simulink model "fbl_4wd_model_debug"  (R2020b)
settings: Solver=VariableStepAuto  StartTime=0.0  StopTime=1  RelTol=1e-6
values from neighbouring files (symbols this model uses):
  a = 0.37    [main.m]
  b = 0.55    [main.m]
  d0 = 0.18    [main.m]
  fr_act = 0.12    [main.m]
  g = 9.81    [main.m]
  I = 20    [main.m]
  M = [m 0 0; 0 m 0; 0 0 I]    [main.m]
  m = 116    [main.m]
  mu_act = 0.88    [main.m]
  q0 = [0;0;deg2rad(10)]    [main.m]
  q0_dot = [[cos(q0(3)) -sin(q0(3));sin(q0(3)) cos(q0(3))]*[0.5;0.5];-2.2]    [main.m]
  r = 0.2    [main.m]
libraries: simulink x2
settings Model: Creator=sumit  LastModifiedBy=sumit

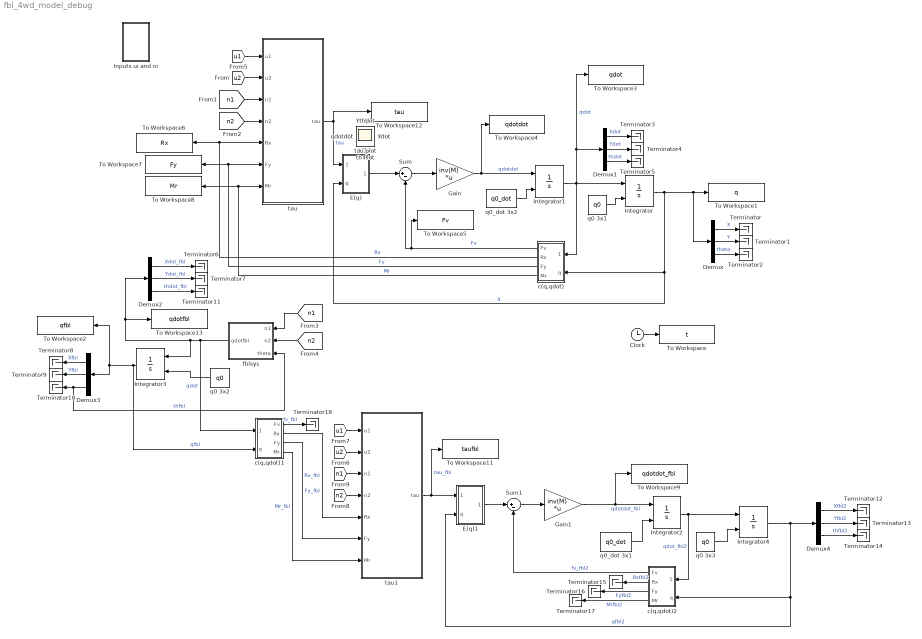
== system fbl_4wd_model_debug ==
  Clock : Clock
  Demux{,1..4} (5 alike) : Demux  Outputs=3
  E(q) : Subsystem
  E(q)1 : Subsystem
  Gain : Gain  Gain=inv(M)  Multiplication=Matrix(K*u) (u vector)
  Gain1 : Gain  Gain=inv(M)  Multiplication=Matrix(K*u) (u vector)
  Inputs ui and ni : Subsystem
  Integrator{,1..4} (5 alike) : Integrator  InitialConditionSource=external
  Sum : Sum  Inputs=|+-
  Sum1 : Sum  Inputs=|+-
  Terminator{,1..18} (19 alike) : Terminator
  To Workspace : ToWorkspace  VariableName=t  SampleTime=-1
  To Workspace1 : ToWorkspace  VariableName=q  SampleTime=-1
  To Workspace11 : ToWorkspace  VariableName=taufbl  SampleTime=-1
  To Workspace12 : ToWorkspace  VariableName=tau  SampleTime=-1
  To Workspace13 : ToWorkspace  VariableName=qdotfbl  SampleTime=-1
  To Workspace2 : ToWorkspace  VariableName=qfbl  SampleTime=-1
  To Workspace3 : ToWorkspace  VariableName=qdot  SampleTime=-1
  To Workspace4 : ToWorkspace  VariableName=qdotdot  SampleTime=-1
  To Workspace5 : ToWorkspace  VariableName=Fv  SampleTime=-1
  To Workspace6 : ToWorkspace  VariableName=Rx  SampleTime=-1
  To Workspace7 : ToWorkspace  VariableName=Fy  SampleTime=-1
  To Workspace8 : ToWorkspace  VariableName=Mr  SampleTime=-1
  To Workspace9 : ToWorkspace  VariableName=qdotdot_fbl  SampleTime=-1
  c(q,qdot) : Subsystem
  c(q,qdot)1 : Subsystem
  c(q,qdot)2 : Subsystem
  fblsys : MATLAB Function  TreatAsAtomicUnit=on
  q0 3x1 : Constant  Value=q0
  q0 3x2 : Constant  Value=q0
  q0 3x3 : Constant  Value=q0
  q0_dot 3x1 : Constant  Value=q0_dot
  q0_dot 3x2 : Constant  Value=q0_dot
  tau : MATLAB Function  TreatAsAtomicUnit=on
  tau1 : MATLAB Function  TreatAsAtomicUnit=on
  Fv : Scope
  Fy : Scope
  Mr : Scope
  Rx : Scope
  X Plot : Scope
  Xdot : Scope
  Y Plot : Scope
  Ydot : Scope
  qdotdot : Scope
  tau plot : Scope
  th Plot : Scope
  thdot : Scope
  wires:
  q0 3x1/1 -> Integrator/2
  q0_dot 3x2/1 -> Integrator1/2
  Gain/1 -> To Workspace4/1, Integrator1/1  "qdotdot"
  Clock/1 -> To Workspace/1
  Integrator/1 -> c(q,qdot)/2(q), E(q)/2(q), Demux/1, To Workspace1/1  "q"
  Sum/1 -> Gain/1
  c(q,qdot)/1(Fv) -> To Workspace5/1, Sum/2  "Fv"
  E(q)/1(Ftau) -> Sum/1
  Demux/1 -> Terminator/1  "X"
  Demux/2 -> Terminator1/1  "Y"
  Demux/3 -> Terminator2/1  "theta"
  Demux1/2 -> Terminator4/1  "Ydot"
  Integrator1/1 -> Integrator/1, c(q,qdot)/1(qdot), To Workspace3/1, Demux1/1  "qdot"
  Demux1/3 -> Terminator5/1  "thdot"
  Demux1/1 -> Terminator3/1  "Xdot"
  tau/1(tau) -> E(q)/1(tau), To Workspace12/1  "tau"
  c(q,qdot)/4(Mr) -> To Workspace8/1, tau/7(Mr)  "Mr"
  c(q,qdot)/3(Fy) -> To Workspace7/1, tau/6(Fy)  "Fy"
  c(q,qdot)/2(Rx) -> To Workspace6/1, tau/5(Rx)  "Rx"
  [n1] -> tau/3(n1)
  [n2] -> tau/4(n2)
  [n1] -> fblsys/1(n1)
  [n2] -> fblsys/2(n2)
  q0 3x2/1 -> Integrator3/2
  Demux3/1 -> Terminator8/1  "Xfbl"
  Integrator3/1 -> c(q,qdot)1/2(q), Demux3/1, To Workspace2/1  "qfbl"
  Demux3/2 -> Terminator9/1  "Yfbl"
  Demux3/3 -> fblsys/3(theta), Terminator10/1  "thfbl"
  Demux2/1 -> Terminator6/1  "Xdot_fbl"
  Demux2/2 -> Terminator7/1  "Ydot_fbl"
  Demux2/3 -> Terminator11/1  "thdot_fbl"
  fblsys/1(qdotfbl) -> Integrator3/1, To Workspace13/1, Demux2/1, c(q,qdot)1/1(qdot)  "qdot"
  c(q,qdot)1/1(Fv) -> Terminator18/1  "fv_fbl"
  c(q,qdot)1/2(Rx) -> tau1/5(Rx)  "Rx_fbl"
  c(q,qdot)1/3(Fy) -> tau1/6(Fy)  "Fy_fbl"
  c(q,qdot)1/4(Mr) -> tau1/7(Mr)  "Mr_fbl"
  [u2] -> tau/2(u2)
  [u1] -> tau/1(u1)
  [u1] -> tau1/1(u1)
  [u2] -> tau1/2(u2)
  [n1] -> tau1/3(n1)
  [n2] -> tau1/4(n2)
  tau1/1(tau) -> To Workspace11/1, E(q)1/1(tau)  "tau_fbl"
  E(q)1/1(Ftau) -> Sum1/1
  Sum1/1 -> Gain1/1
  Gain1/1 -> Integrator2/1, To Workspace9/1  "qdotdot_fbl"
  q0_dot 3x1/1 -> Integrator2/2
  q0 3x3/1 -> Integrator4/2
  Integrator2/1 -> Integrator4/1, c(q,qdot)2/1(qdot)  "qdot_fbl2"
  Integrator4/1 -> E(q)1/2(q), c(q,qdot)2/2(q), Demux4/1  "qfbl2"
  Demux4/1 -> Terminator12/1  "Xfbl2"
  Demux4/2 -> Terminator13/1  "Yfbl2"
  Demux4/3 -> Terminator14/1  "thfbl2"
  c(q,qdot)2/2(Rx) -> Terminator15/1  "Rxfbl2"
  c(q,qdot)2/3(Fy) -> Terminator16/1  "Fyfbl2"
  c(q,qdot)2/4(Mr) -> Terminator17/1  "Mrfbl2"
  c(q,qdot)2/1(Fv) -> Sum1/2  "fv_fbl2"

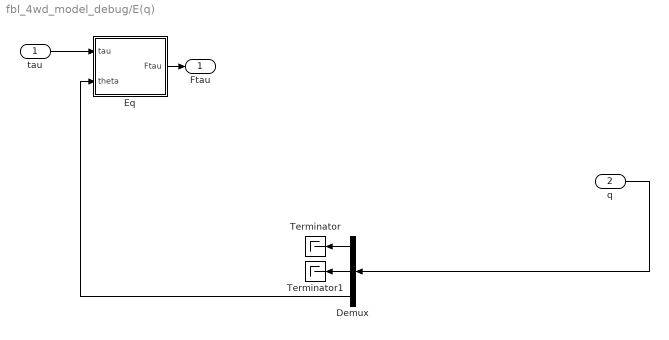
== system fbl_4wd_model_debug/E(q) ==
  tau : Inport
  q : Inport  Port=2
  Demux : Demux  Outputs=3
  Eq : MATLAB Function  TreatAsAtomicUnit=on
  Terminator : Terminator
  Terminator1 : Terminator
  Ftau : Outport
  wires:
  Demux/1 -> Terminator/1
  Eq/1(Ftau) -> Ftau/1
  q/1 -> Demux/1
  Demux/2 -> Terminator1/1
  tau/1 -> Eq/1(tau)
  Demux/3 -> Eq/2(theta)

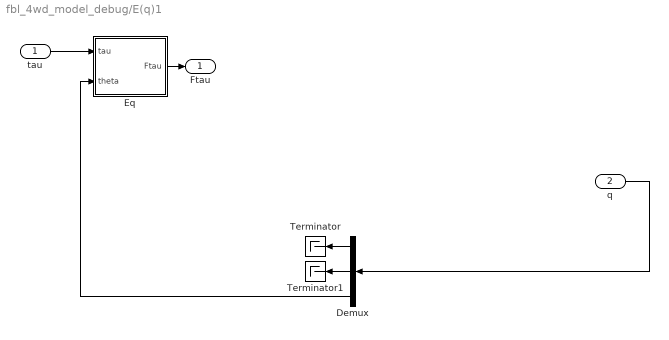
== system fbl_4wd_model_debug/E(q)1 ==
  tau : Inport
  q : Inport  Port=2
  Demux : Demux  Outputs=3
  Eq : MATLAB Function  TreatAsAtomicUnit=on
  Terminator : Terminator
  Terminator1 : Terminator
  Ftau : Outport
  wires:
  Demux/1 -> Terminator/1
  Eq/1(Ftau) -> Ftau/1
  q/1 -> Demux/1
  Demux/2 -> Terminator1/1
  tau/1 -> Eq/1(tau)
  Demux/3 -> Eq/2(theta)

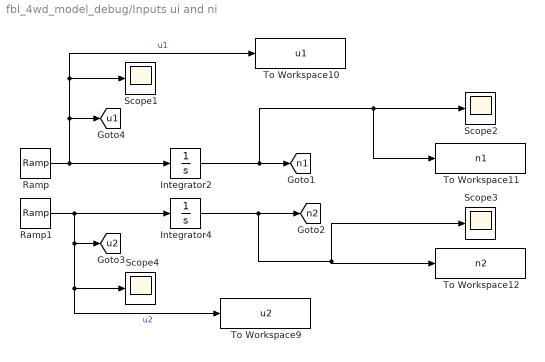
== system fbl_4wd_model_debug/Inputs ui and ni ==
  Integrator2 : Integrator
  Integrator4 : Integrator
  Ramp : simulink/Sources/Ramp  slope=0.5  start=0.2  InitialOutput=0
  Ramp1 : simulink/Sources/Ramp  slope=1  start=0.2  InitialOutput=0
  Scope{1..4} (4 alike) : Scope
  To Workspace10 : ToWorkspace  VariableName=u1  SampleTime=-1
  To Workspace11 : ToWorkspace  VariableName=n1  SampleTime=-1
  To Workspace12 : ToWorkspace  VariableName=n2  SampleTime=-1
  To Workspace9 : ToWorkspace  VariableName=u2  SampleTime=-1
  tag scope: n1=global, n2=global, u1=global, u2=global
  wires:
  Ramp1/1 -> Integrator4/1, [u2], To Workspace9/1, Scope4/1  "u2"
  Ramp/1 -> Integrator2/1, [u1], To Workspace10/1, Scope1/1  "u1"
  Integrator4/1 -> Scope3/1, To Workspace12/1, [n2]
  Integrator2/1 -> To Workspace11/1, Scope2/1, [n1]

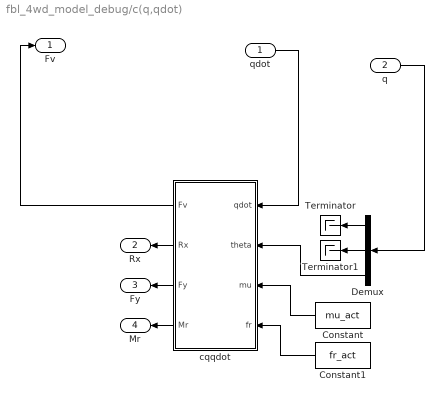
== system fbl_4wd_model_debug/c(q,qdot) ==
  qdot : Inport
  q : Inport  Port=2
  Constant : Constant  Value=mu_act
  Constant1 : Constant  Value=fr_act
  Demux : Demux  Outputs=3
  Terminator : Terminator
  Terminator1 : Terminator
  cqqdot : MATLAB Function  TreatAsAtomicUnit=on
  Fv : Outport
  Rx : Outport  Port=2
  Fy : Outport  Port=3
  Mr : Outport  Port=4
  wires:
  Demux/2 -> Terminator1/1
  cqqdot/1(Fv) -> Fv/1
  qdot/1 -> cqqdot/1(qdot)
  Constant1/1 -> cqqdot/4(fr)
  Demux/1 -> Terminator/1
  Constant/1 -> cqqdot/3(mu)
  Demux/3 -> cqqdot/2(theta)
  q/1 -> Demux/1
  cqqdot/3(Fy) -> Fy/1
  cqqdot/2(Rx) -> Rx/1
  cqqdot/4(Mr) -> Mr/1

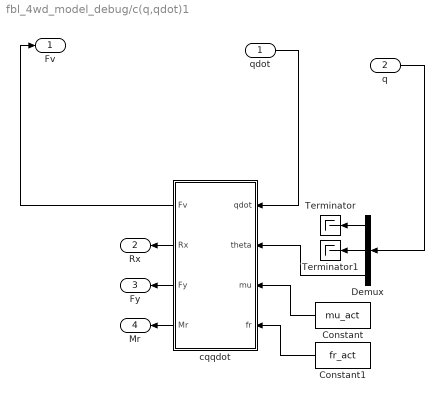
== system fbl_4wd_model_debug/c(q,qdot)1 ==
  qdot : Inport
  q : Inport  Port=2
  Constant : Constant  Value=mu_act
  Constant1 : Constant  Value=fr_act
  Demux : Demux  Outputs=3
  Terminator : Terminator
  Terminator1 : Terminator
  cqqdot : MATLAB Function  TreatAsAtomicUnit=on
  Fv : Outport
  Rx : Outport  Port=2
  Fy : Outport  Port=3
  Mr : Outport  Port=4
  wires:
  Demux/2 -> Terminator1/1
  cqqdot/1(Fv) -> Fv/1
  qdot/1 -> cqqdot/1(qdot)
  Constant1/1 -> cqqdot/4(fr)
  Demux/1 -> Terminator/1
  Constant/1 -> cqqdot/3(mu)
  Demux/3 -> cqqdot/2(theta)
  q/1 -> Demux/1
  cqqdot/3(Fy) -> Fy/1
  cqqdot/2(Rx) -> Rx/1
  cqqdot/4(Mr) -> Mr/1

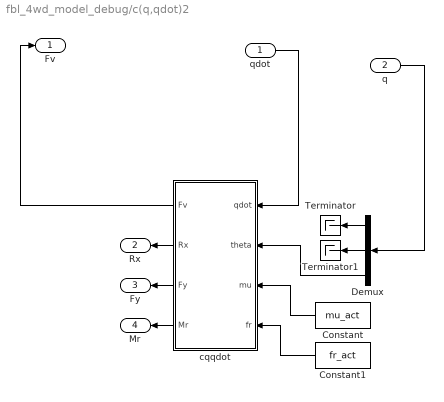
== system fbl_4wd_model_debug/c(q,qdot)2 ==
  qdot : Inport
  q : Inport  Port=2
  Constant : Constant  Value=mu_act
  Constant1 : Constant  Value=fr_act
  Demux : Demux  Outputs=3
  Terminator : Terminator
  Terminator1 : Terminator
  cqqdot : MATLAB Function  TreatAsAtomicUnit=on
  Fv : Outport
  Rx : Outport  Port=2
  Fy : Outport  Port=3
  Mr : Outport  Port=4
  wires:
  Demux/2 -> Terminator1/1
  cqqdot/1(Fv) -> Fv/1
  qdot/1 -> cqqdot/1(qdot)
  Constant1/1 -> cqqdot/4(fr)
  Demux/1 -> Terminator/1
  Constant/1 -> cqqdot/3(mu)
  Demux/3 -> cqqdot/2(theta)
  q/1 -> Demux/1
  cqqdot/3(Fy) -> Fy/1
  cqqdot/2(Rx) -> Rx/1
  cqqdot/4(Mr) -> Mr/1

== matlab function fbl_4wd_model_debug/E(q)1/Eq ==
  data: tau input; theta input; Ftau output; t parameter; r parameter
function Ftau = Eq(tau,theta,t, r)
Ftau=[cos(theta)/r cos(theta)/r;...
   sin(theta)/r sin(theta)/r;...
   -t/r t/r]*tau;

== matlab function fbl_4wd_model_debug/c(q,qdot)2/cqqdot ==
  data: qdot input; theta input; Fv output; mu input; fr input; a parameter; b parameter; t parameter; g parameter; m parameter; Rx output; Fy output; Mr output
function [Fv,Rx,Fy,Mr] = cqqdot(qdot,theta,mu,fr,a, b, t, g, m)
Xdot=qdot(1);
Ydot=qdot(2);
thdot=qdot(3);

%Rth = [cos(theta) -sin(theta);sin(theta) cos(theta)];

xdot =  Xdot*cos(theta)+Ydot*sin(theta);
ydot = -Xdot*sin(theta)+Ydot*cos(theta);

x1dot = xdot-t*thdot;   
x2dot = xdot+t*thdot;
y1dot = ydot+a*thdot;
y3dot = ydot-b*thdot;

% Rx = fr*m*g*0.5*(sign(round(x1dot))+sign(round(x2dot)));
% Fy = mu*m*g*(b*sign(round(y1dot,5))+a*sign(round(y3dot,5)))/(a+b);
% Mr = mu*a*b*m*g*(sign(round(y1dot,5))-sign(round(y3dot,5)))/(a+b)...
%      + fr*t*m*g*0.5*(sign(round(x2dot,5))-sign(round(x1dot,5)));
Rx = fr*m*g*0.5*(sign(x1dot)+sign(x2dot));
Fy = mu*m*g*(b*sign(y1dot)+a*sign(y3dot))/(a+b);
Mr = mu*a*b*m*g*(sign(y1dot)-sign(y3dot))/(a+b)...
     + fr*t*m*g*0.5*(sign(x2dot)-sign(x1dot));
 
Fv=[Rx*cos(theta)-Fy*sin(theta);...
   Rx*sin(theta)+Fy*cos(theta);...
   Mr];

== matlab function fbl_4wd_model_debug/E(q)/Eq ==
  data: tau input; theta input; Ftau output; t parameter; r parameter
function Ftau = Eq(tau,theta,t, r)
Ftau=[cos(theta)/r cos(theta)/r;...
   sin(theta)/r sin(theta)/r;...
   -t/r t/r]*tau;

== matlab function fbl_4wd_model_debug/c(q,qdot)/cqqdot ==
  data: qdot input; theta input; Fv output; mu input; fr input; a parameter; b parameter; t parameter; g parameter; m parameter; Rx output; Fy output; Mr output
function [Fv,Rx,Fy,Mr] = cqqdot(qdot,theta,mu,fr,a, b, t, g, m)
Xdot=qdot(1);
Ydot=qdot(2);
thdot=qdot(3);

%Rth = [cos(theta) -sin(theta);sin(theta) cos(theta)];

xdot =  Xdot*cos(theta)+Ydot*sin(theta);
ydot = -Xdot*sin(theta)+Ydot*cos(theta);

x1dot = xdot-t*thdot;   
x2dot = xdot+t*thdot;
y1dot = ydot+a*thdot;
y3dot = ydot-b*thdot;

Rx = fr*m*g*0.5*(sign(x1dot)+sign(x2dot));
Fy = mu*m*g*(b*sign(y1dot)+a*sign(y3dot))/(a+b);
Mr = mu*a*b*m*g*(sign(y1dot)-sign(y3dot))/(a+b)...
     + fr*t*m*g*0.5*(sign(x2dot)-sign(x1dot));
 
Fv=[Rx*cos(theta)-Fy*sin(theta);...
   Rx*sin(theta)+Fy*cos(theta);...
   Mr];

== matlab function fbl_4wd_model_debug/tau ==
  data: u1 input; u2 input; n1 input; n2 input; Rx input; Fy input; Mr input; tau output; t parameter; r parameter; d0 parameter; m parameter; I parameter
function tau = FBL(u1,u2,n1,n2,Rx,Fy,Mr,t, r,d0, m, I)
tau=[r*0.5*(m*u1+m*n2*n2/d0+Rx)+(r*d0*0.5/t)*((m+I/(d0^2))*u2-m*n1*n2/d0...
    +Fy-Mr/d0);
     r*0.5*(m*u1+m*n2*n2/d0+Rx)-(r*d0*0.5/t)*((m+I/(d0^2))*u2-m*n1*n2/d0...
    +Fy-Mr/d0)];

== matlab function fbl_4wd_model_debug/fblsys ==
  data: n1 input; n2 input; theta input; qdotfbl output; d0 parameter
function qdotfbl = fblsys(n1, n2,theta,d0)
qdotfbl=[cos(theta)*n1-sin(theta)*n2;...
         sin(theta)*n1+cos(theta)*n2;...
         -n2/d0];

== matlab function fbl_4wd_model_debug/c(q,qdot)1/cqqdot ==
  data: qdot input; theta input; Fv output; mu input; fr input; a parameter; b parameter; t parameter; g parameter; m parameter; Rx output; Fy output; Mr output
function [Fv,Rx,Fy,Mr] = cqqdot(qdot,theta,mu,fr,a, b, t, g, m)
Xdot=qdot(1);
Ydot=qdot(2);
thdot=qdot(3);

%Rth = [cos(theta) -sin(theta);sin(theta) cos(theta)];

xdot =  Xdot*cos(theta)+Ydot*sin(theta);
ydot = -Xdot*sin(theta)+Ydot*cos(theta);

x1dot = xdot-t*thdot;   
x2dot = xdot+t*thdot;
y1dot = ydot+a*thdot;
y3dot = ydot-b*thdot;

Rx = fr*m*g*0.5*(sign(x1dot)+sign(x2dot));
Fy = mu*m*g*(b*sign(y1dot)+a*sign(y3dot))/(a+b);
Mr = mu*a*b*m*g*(sign(y1dot)-sign(y3dot))/(a+b)...
     + fr*t*m*g*0.5*(sign(x2dot)-sign(x1dot));
 
Fv=[Rx*cos(theta)-Fy*sin(theta);...
   Rx*sin(theta)+Fy*cos(theta);...
   Mr];

== matlab function fbl_4wd_model_debug/tau1 ==
  data: u1 input; u2 input; n1 input; n2 input; Rx input; Fy input; Mr input; tau output; t parameter; r parameter; d0 parameter; m parameter; I parameter
function tau = FBL(u1,u2,n1,n2,Rx,Fy,Mr,t, r,d0, m, I)
tau=[r*0.5*(m*u1+m*n2*n2/d0+Rx)+(r*d0*0.5/t)*((m+I/(d0^2))*u2-m*n1*n2/d0...
    +Fy-Mr/d0);
     r*0.5*(m*u1+m*n2*n2/d0+Rx)-(r*d0*0.5/t)*((m+I/(d0^2))*u2-m*n1*n2/d0...
    +Fy-Mr/d0)];
